simulink model "robustMPC_getInput_sim"  (R2013a)
settings: Solver=ode45  StartTime=0.0  StopTime=10.0  RelTol=1e-3
settings Model: Creator=Kostas  LastModifiedBy=Kostas

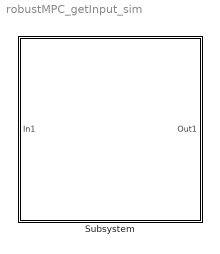
== system robustMPC_getInput_sim ==
  Subsystem : Subsystem

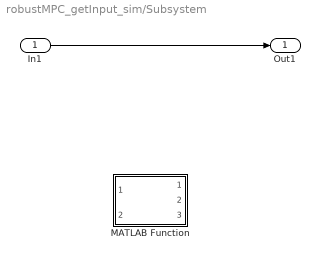
== system robustMPC_getInput_sim/Subsystem ==
  In1 : Inport
  MATLAB Function : MATLAB Function  TreatAsAtomicUnit=on
  Out1 : Outport
  wires:
  In1/1 -> Out1/1

== matlab function robustMPC_getInput_sim/Subsystem/MATLAB Function ==
  data: x_state_value input; u_ctrl_out output; sol_x_mp input; sol_found_out output; flag_strange_out output
function [u_ctrl_out,sol_found_out,flag_strange_out] = robustMPC_getInput_sim(x_state_value,sol_x_mp)

[u_ctrl,sol_found, flag_strange] = robustmpc_getInput(sol_x_mp, x_state_value);

u_ctrl_out = u_ctrl;
sol_found_out = sol_found;
flag_strange_out = flag_strange;

end
